simulink model "stabilizacja_pid_rownolegle"  (R2013b)
settings: Solver=ode4  StartTime=0.0  StopTime=tSim  FixedStep=h  RelTol=1e-3
values from neighbouring files (symbols this model uses):
  Kp1 = -50.8    [launcher_simulink.m]
  Kp2 = 6    [launcher_simulink.m]
  modelSelect = 'full'    [launcher_script.m]    (also in launcher_simulink.m = 'linear')
  params = [M,m,L,I,b,g]    [launcher_script.m]    (also in launcher_simulink.m)
  state0 = [thetaDot0;theta0;xDot0;x0]    [launcher_script.m]    (also in launcher_simulink.m; sFunction.m = [])
  Td1 = 0.24    [launcher_simulink.m]
  Td2 = 1.5    [launcher_simulink.m]
  Ti1 = 7.26    [launcher_simulink.m]
  Ti2 = inf    [launcher_simulink.m]
settings Model: Creator=JAR  LastModifiedBy=JAR

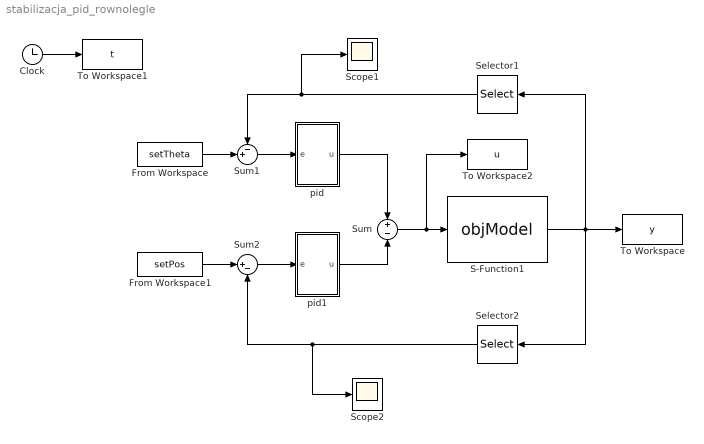
== system stabilizacja_pid_rownolegle ==
  Clock : Clock
  From Workspace : FromWorkspace  VariableName=setTheta  SampleTime=0
  From Workspace1 : FromWorkspace  VariableName=setPos  SampleTime=0
  S-Function1 : S-Function  FunctionName=objModel  Parameters=state0,params,modelSelect  EnableBusSupport=off
  Scope1 : Scope
  Scope2 : Scope
  Selector1 : Selector  InputPortWidth=4  IndexOptions=Index vector (dialog)  Indices=2  OutputSizes=1
  Selector2 : Selector  InputPortWidth=4  IndexOptions=Index vector (dialog)  Indices=4  OutputSizes=1
  Sum : Sum  Inputs=+-
  Sum1 : Sum  Inputs=-+|
  Sum2 : Sum  Inputs=|+-
  To Workspace : ToWorkspace  VariableName=y  SampleTime=-1
  To Workspace1 : ToWorkspace  VariableName=t  SampleTime=-1
  To Workspace2 : ToWorkspace  VariableName=u  SampleTime=-1
  pid : Subsystem
  pid1 : Subsystem
  wires:
  S-Function1/1 -> Selector1/1, Selector2/1, To Workspace/1
  Clock/1 -> To Workspace1/1
  pid/1(u) -> Sum/1
  pid1/1(u) -> Sum/2
  Sum/1 -> To Workspace2/1, S-Function1/1
  From Workspace/1 -> Sum1/2
  Sum1/1 -> pid/1(e)
  Selector1/1 -> Scope1/1, Sum1/1
  Sum2/1 -> pid1/1(e)
  Selector2/1 -> Scope2/1, Sum2/2
  From Workspace1/1 -> Sum2/1

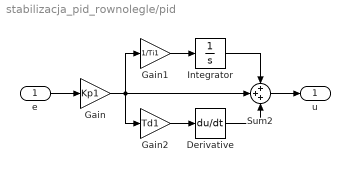
== system stabilizacja_pid_rownolegle/pid ==
  e : Inport
  Derivative : Derivative
  Gain : Gain  Gain=Kp1
  Gain1 : Gain  Gain=1/Ti1
  Gain2 : Gain  Gain=Td1
  Integrator : Integrator
  Sum2 : Sum  Inputs=+++
  u : Outport
  wires:
  Sum2/1 -> u/1
  Gain1/1 -> Integrator/1
  Gain/1 -> Gain2/1, Gain1/1, Sum2/2
  e/1 -> Gain/1
  Derivative/1 -> Sum2/3
  Integrator/1 -> Sum2/1
  Gain2/1 -> Derivative/1

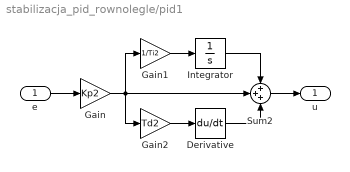
== system stabilizacja_pid_rownolegle/pid1 ==
  e : Inport
  Derivative : Derivative
  Gain : Gain  Gain=Kp2
  Gain1 : Gain  Gain=1/Ti2
  Gain2 : Gain  Gain=Td2
  Integrator : Integrator
  Sum2 : Sum  Inputs=+++
  u : Outport
  wires:
  Sum2/1 -> u/1
  Gain1/1 -> Integrator/1
  Gain/1 -> Gain2/1, Gain1/1, Sum2/2
  e/1 -> Gain/1
  Derivative/1 -> Sum2/3
  Integrator/1 -> Sum2/1
  Gain2/1 -> Derivative/1
